simulink model "lunchline_ex4"  (R2016a)
settings: Solver=VariableStepAuto  StartTime=0.0  StopTime=90  RelTol=1e-3
undefined symbols (not defined in the file or in its folder): m, n
settings Model: Creator=ningd  LastModifiedBy=ningd

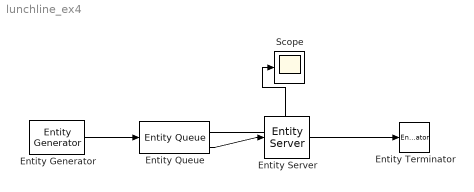
== system lunchline_ex4 ==
  Entity Generator : EntityGenerator  OutputPortMessageModes=m  TimeSource=MATLAB action  IntergenerationTimeAction=dt = exprnd(0.5);  GenerateEntityAtSimulationStart=off  GenerateAction=|  AttributeName=ServiceTime  EntityType=Structured  EntityTypeName=Customer
      | % Define a service time from a normal distribution 
      | % with mean 1.7 and std deviation 0.2
      | entity.ServiceTime = 1.7 + 0.2*randn;
  Entity Queue : EntityQueue  InputPortMessageModes=m  OutputPortMessageModes=n,m  NumberEntitiesInBlock=on
      settings: OutputPortMap=o1,o5
  Entity Server : EntityServer  InputPortMessageModes=m  OutputPortMessageModes=m  Capacity=2  ServiceTimeSource=Attribute
  Entity Terminator : EntityTerminator  InputPortMessageModes=m
  Scope : Scope
  wires:
  Entity Generator/1 -> Entity Queue/1
  Entity Queue/2 -> Entity Server/1
  Entity Server/1 -> Entity Terminator/1
  Entity Queue/1 -> Scope/1
